simulink model "MSAP"  (R2023b)
settings: Solver=VariableStepAuto  StartTime=0.0  StopTime=10  RelTol=1e-3
undefined symbols (not defined in the file): A1, A2, B1, B2, F, Fie, J, Ld, Lq, P, Rs
libraries: slpidlib x1
settings Model: Creator=lylia  LastModifiedBy=lylia

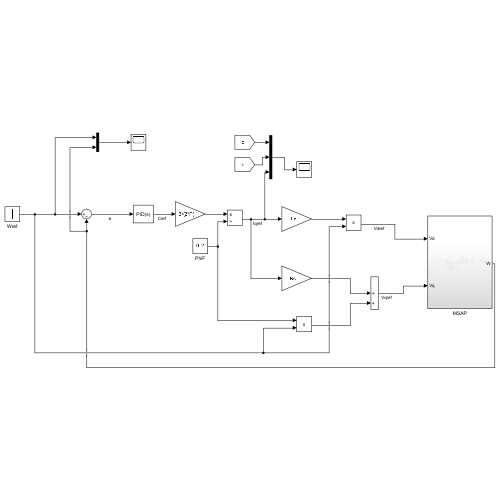
[thumbnail: Simulink's stored preview of the top-level diagram]
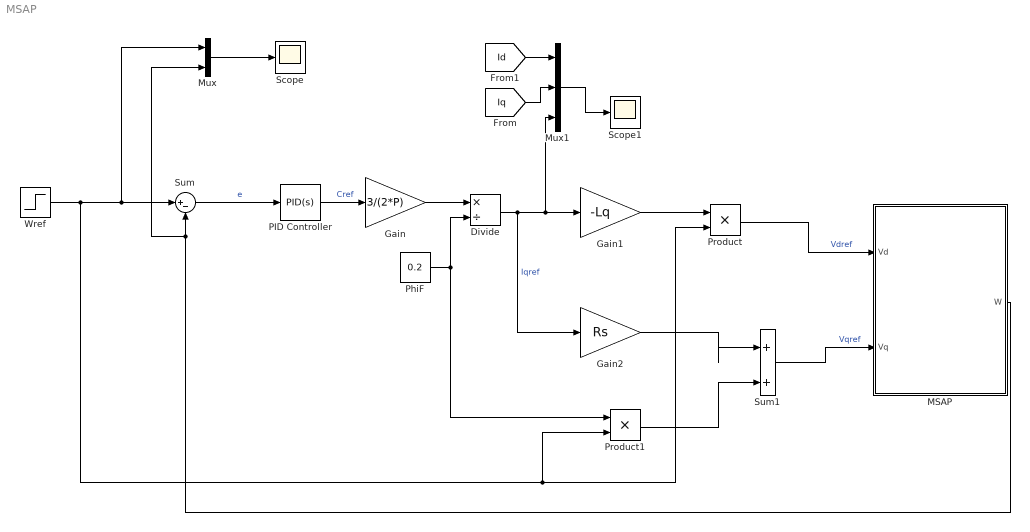
== system MSAP ==
  Divide : Product  Inputs=*/
  Gain : Gain  Gain=3/(2*P)
  Gain1 : Gain  Gain=-Lq
  Gain2 : Gain  Gain=Rs
  MSAP : Subsystem
  Mux : Mux  Inputs=2
  Mux1 : Mux  Inputs=3
  PID Controller : slpidlib/PID Controller  Controller=PID  Form=Parallel  TimeDomain=Continuous-time  UseExternalTs=off  SampleTime=-1  IntegratorMethod=Forward Euler  FilterMethod=Forward Euler  ControllerParametersSource=internal  P=0.1  I=0.5  UseKiTs=off  D=0  N=100  UseFilter=on  TunerSelectOption=Transfer Function Based (PID Tuner App)  InitialConditionSource=internal  InitialConditionForIntegrator=0  InitialConditionForFilter=0  DifferentiatorICPrevScaledInput=0  ExternalReset=none  TrackingMode=off  Kt=1  LimitOutput=off  SatLimitsSource=internal  UpperSaturationLimit=inf  LowerSaturationLimit=-inf  LinearizeAsGain=on  AntiWindupMode=none  Kb=1  LimitIntegrator=off  UpperIntegratorSaturationLimit=inf  LowerIntegratorSaturationLimit=-inf  POutMin=[]  POutMax=[]  IOutMin=[]  IOutMax=[]  DOutMin=[]  DOutMax=[]  NOutMin=[]  NOutMax=[]  SumOutMin=[]  SumOutMax=[]  SaturationOutMin=[]  SaturationOutMax=[]  PParamMin=[]  PParamMax=[]  IParamMin=[]  IParamMax=[]  DParamMin=[]  DParamMax=[]  NParamMin=[]  NParamMax=[]  KbParamMin=[]  KbParamMax=[]  KtParamMin=[]  KtParamMax=[]  KbOutMin=[]  KbOutMax=[]  KtOutMin=[]  KtOutMax=[]  IntegratorOutMin=[]  IntegratorOutMax=[]  FilterOutMin=[]  FilterOutMax=[]  SumI1OutMin=[]  SumI1OutMax=[]  SumI2OutMin=[]  SumI2OutMax=[]  SumI3OutMin=[]  SumI3OutMax=[]  SumI4OutMin=[]  SumI4OutMax=[]  SumDOutMin=[]  SumDOutMax=[]  DifferentiatorOutMin=[]  DifferentiatorOutMax=[]  FilterDiffOutCoefMin=[]  FilterDiffOutCoefMax=[]  ReciprocalOutMin=[]  ReciprocalOutMax=[]  SumDenOutMin=[]  SumDenOutMax=[]  SumNumOutMin=[]  SumNumOutMax=[]  DivideOutMin=[]  DivideOutMax=[]  UdiffTsProdOutMin=[]  UdiffTsProdOutMax=[]  NTsProdOutMin=[]  NTsProdOutMax=[]  UintegralTsProdOutMin=[]  UintegralTsProdOutMax=[]  UngainTsProdOutMin=[]  UngainTsProdOutMax=[]  ClampingZeroOutDataTypeStr=Inherit: Inherit via back propagation  ClampingZeroOutMin=[]  ClampingZeroOutMax=[]  FilterDenConstantOutDataTypeStr=Inherit: Inherit via back propagation  FilterDenConstantOutMin=[]  FilterDenConstantOutMax=[]  PCopyOutDataTypeStr=Inherit: Inherit via back propagation  PCopyOutMin=[]  PCopyOutMax=[]  NCopyOutDataTypeStr=Inherit: Inherit via back propagation  NCopyOutMin=[]  NCopyOutMax=[]  IntegratorContinuousStateAttributes=''  IntegratorStateMustResolveToSignalObject=off  IntegratorRTWStateStorageClass=Auto  FilterContinuousStateAttributes=''  FilterStateMustResolveToSignalObject=off  FilterRTWStateStorageClass=Auto  ParallelPVariant=InternalParameters  IdealPVariant=Disabled  IVariant=InternalParameters  DVariant=InternalParameters  IntegratorVariant=Continuous  SatVariant=Disabled  AWVariant=Passthrough  PCopyVariant=Disabled  TRVariant=Disabled  FdbkBlocksVariant=Forward  IdealPFdbkVariant=Disabled  SatFdbkVariant=Disabled  DerivativeFilterVariant=ContFilter  NVariant=InternalParameters  NCopyVariant=Disabled  FilterICVariant=InternalICsFilter  IntegratorICVariant=InternalICs  ExternalResetVariant=Disabled  TRSumVariant=Passthrough  SumFdbkVariant=Disabled  SumVariant=Sum_PID  TsampFilterVariant=InternalTs  TsampNgainVariant=Passthrough  TsampIntegralVariant=Disabled_SignalSpec  ExternalSaturationOutDataTypeStr=Inherit: Same as second input
  PhiF : Constant  Value=0.2
  Product : Product
  Product1 : Product
  Scope : Scope
  Scope1 : Scope
  Sum : Sum  Inputs=|+-
  Sum1 : Sum  Inputs=|++
  Wref : Step  Time=3  Before=2*pi*50  After=2*pi*75  SampleTime=0
  wires:
  MSAP/1(W) -> Mux/2, Sum/2
  Sum/1 -> PID Controller/1  "e"
  PID Controller/1 -> Gain/1  "Cref"
  Gain/1 -> Divide/1
  PhiF/1 -> Product1/1, Divide/2
  Divide/1 -> Gain2/1, Mux1/3, Gain1/1  "Iqref"
  Gain1/1 -> Product/1
  Wref/1 -> Product1/2, Product/2, Mux/1, Sum/1
  Gain2/1 -> Sum1/1
  Product1/1 -> Sum1/2
  Sum1/1 -> MSAP/2(Vq)  "Vqref"
  Product/1 -> MSAP/1(Vd)  "Vdref"
  Mux/1 -> Scope/1
  Mux1/1 -> Scope1/1
  [Iq] -> Mux1/2
  [Id] -> Mux1/1

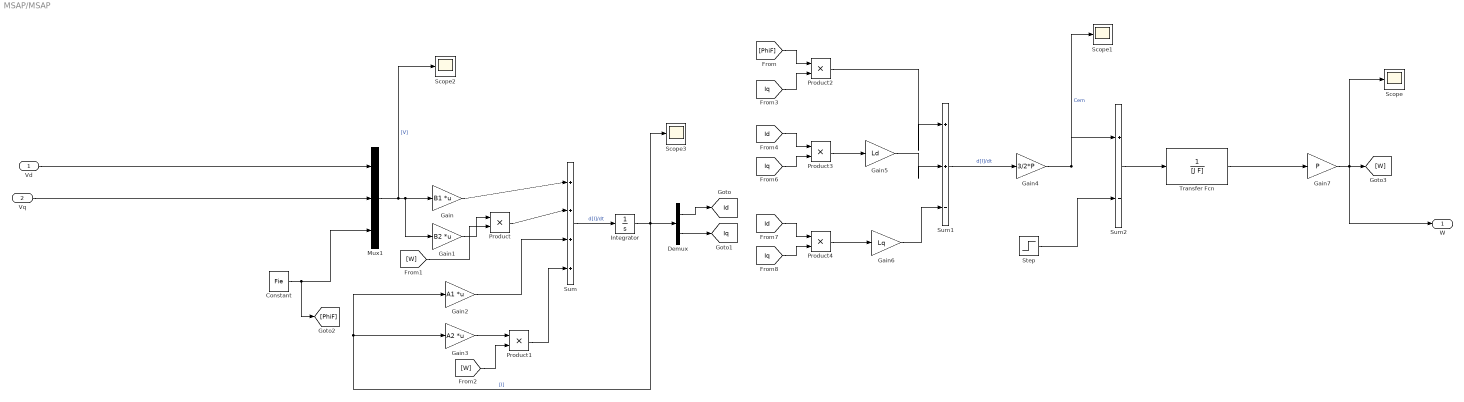
== system MSAP/MSAP ==
  Vd : Inport
  Vq : Inport  Port=2
  Constant : Constant  Value=Fie
  Demux : Demux  Outputs=2
  Gain : Gain  Gain=B1  Multiplication=Matrix(K*u)
  Gain1 : Gain  Gain=B2  Multiplication=Matrix(K*u)
  Gain2 : Gain  Gain=A1  Multiplication=Matrix(K*u)
  Gain3 : Gain  Gain=A2  Multiplication=Matrix(K*u)
  Gain4 : Gain  Gain=3/2*P
  Gain5 : Gain  Gain=Ld
  Gain6 : Gain  Gain=Lq
  Gain7 : Gain  Gain=P
  Integrator : Integrator
  Mux1 : Mux  Inputs=3
  Product{,1..4} (5 alike) : Product
  Scope{,1..3} (4 alike) : Scope
  Step : Step  Time=5  Before=0.5  After=3  SampleTime=0
  Sum : Sum  Inputs=|++++
  Sum1 : Sum  Inputs=|++-
  Sum2 : Sum  Inputs=|+-
  Transfer Fcn : TransferFcn  Denominator=[J F]
  W : Outport
  tag scope: Id=global, Iq=global
  wires:
  Gain2/1 -> Sum/3
  Mux1/1 -> Scope2/1, Gain1/1, Gain/1  "[V]"
  Constant/1 -> [PhiF], Mux1/3
  Gain/1 -> Sum/1
  Product/1 -> Sum/2
  Integrator/1 -> Gain3/1, Gain2/1, Scope3/1, Demux/1  "[I]"
  Sum2/1 -> Transfer Fcn/1
  Gain1/1 -> Product/1
  Demux/2 -> [Iq]
  Gain7/1 -> W/1, Scope/1, [W]
  Product1/1 -> Sum/4
  Vd/1 -> Mux1/1
  Demux/1 -> [Id]
  [Id] -> Product3/1
  Product2/1 -> Sum1/1
  Product3/1 -> Gain5/1
  Gain5/1 -> Sum1/2
  [Iq] -> Product4/2
  [PhiF] -> Product2/1
  Gain6/1 -> Sum1/3
  [W] -> Product1/2
  [Iq] -> Product2/2
  [W] -> Product/2
  Vq/1 -> Mux1/2
  Product4/1 -> Gain6/1
  [Id] -> Product4/1
  Sum1/1 -> Gain4/1  "d[I]/dt"
  Step/1 -> Sum2/2
  Gain4/1 -> Scope1/1, Sum2/1  "Cem"
  [Iq] -> Product3/2
  Gain3/1 -> Product1/1
  Transfer Fcn/1 -> Gain7/1
  Sum/1 -> Integrator/1  "d[I]/dt"
